simulink model "ecualizador"  (R2017b)
settings: Solver=VariableStepAuto  StartTime=0.0  StopTime=3  RelTol=1e-3
values from neighbouring files (symbols this model uses):
  ganancia = [.001 4 8 2 .1]    [DSP4.m]
  ts = 11025    [DSP4.m]
libraries: dspvision x1
settings Model: Creator=Agustin  LastModifiedBy=Agustin

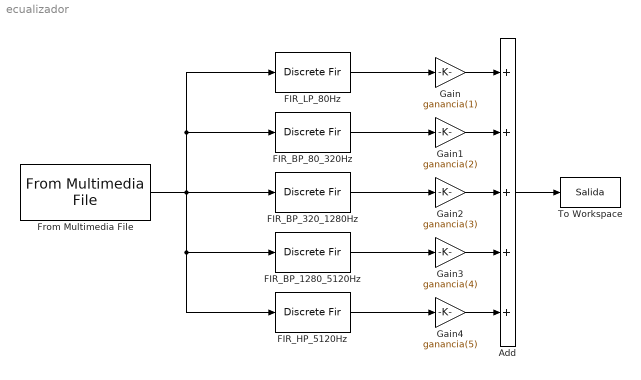
== system ecualizador ==
  Add : Sum  Inputs=+++++
  FIR_BP_1280_5120Hz : DiscreteFir  Tag=BlockMethodSubSystem  Coefficients=[-6.33540936235722367e-05 0.00195654270160462588 -4.01545452605399819e-05 0.00212945592350992276 -0.00285797352861382739 0.000192733862020878858 -0.00635868238869501546 0.00104177495203475841 -0.00246690417021121124 0.00822982232945761866 0.00663127303390260558 0.00720161481872818015 0.0036235549914843063 -0.0160254810773749479 -0.00644133758605169252 -0.0354313467654868985 0.0162538806667236642 -0.0169878821534266526 0.0727785965575659527 -0.00137886733993559853 0.0802568846706619293 -0.0750914551527820662 -0.0198348370109410477 -0.223435374456706137 -0.140838210653331991 0.695680638093415515 -0.140838210653331991 -0.223435374456706137 -0.0198348370109410477 -0.0750914551527820662 0.0802568846706619293 -0.00137886733993559853 0.0727785965575659527 -0.0169878821534266526 0.0162538806667236642 -0.0354313467654868985 -0.00644133758605169252 -0.0160254810773749479 0.0036235549914843063 0.00720161481872818015 0.00663127303390260558 0.00822982232945761866 -0.00246690417021121124 0.00104177495203475841 -0.00635868238869501546 0.000192733862020878858 -0.00285797352861382739 0.00212945592350992276 -4.01545452605399819e-05 0.00195654270160462588 -6.33540936235722367e-05]  InputProcessing=Columns as channels (frame based)  SampleTime=ts
  FIR_BP_320_1280Hz : DiscreteFir  Tag=BlockMethodSubSystem  Coefficients=[0.000419942512208930948 -3.28988295900055057e-05 -1.08715141066685234e-05 0.000698158881007576726 0.00209982001039358494 0.00368828009137740862 0.00437745590019822991 0.00294020690183505054 -0.00112851569328516698 -0.00684304173297955315 -0.0117374599789034622 -0.0130100060708184962 -0.00942737497665724691 -0.00291200710251219696 0.00142417065446380302 -0.00261072713857117382 -0.0186716075625321248 -0.044528875633302753 -0.0710778113878306611 -0.084908586891173865 -0.0738699802862342741 -0.0332917571410572821 0.0302207698048555275 0.0996866081926109926 0.153492724260163749 0.173735970087244396 0.153492724260163749 0.0996866081926109926 0.0302207698048555275 -0.0332917571410572821 -0.0738699802862342741 -0.084908586891173865 -0.0710778113878306611 -0.044528875633302753 -0.0186716075625321248 -0.00261072713857117382 0.00142417065446380302 -0.00291200710251219696 -0.00942737497665724691 -0.0130100060708184962 -0.0117374599789034622 -0.00684304173297955315 -0.00112851569328516698 0.00294020690183505054 0.00437745590019822991 0.00368828009137740862 0.00209982001039358494 0.000698158881007576726 -1.08715141066685234e-05 -3.28988295900055057e-05 0.000419942512208930948]  InputProcessing=Columns as channels (frame based)  SampleTime=ts
  FIR_BP_80_320Hz : DiscreteFir  Tag=BlockMethodSubSystem  Coefficients=[-0.00334531967217268104 -0.00351971885205419914 -0.00392813756457967289 -0.00452322525656722024 -0.00521978418872912249 -0.00589804359324740384 -0.00641026710657543238 -0.00659034250564381838 -0.00626574065394652508 -0.00527100932474330788 -0.00346180649641677574 -0.00072839160035881507 0.00299250896620734379 0.00770846163075225316 0.0133655445192406037 0.0198466230531161025 0.0269739906190492561 0.0345163619960699164 0.0421998798339282832 0.0497224859255611523 0.056770743735437057 0.0630379979484618491 0.0682426371445713775 0.0721451973109596828 0.0745631099123155588 0.0753820543913198554 0.0745631099123155588 0.0721451973109596828 0.0682426371445713775 0.0630379979484618491 0.056770743735437057 0.0497224859255611523 0.0421998798339282832 0.0345163619960699164 0.0269739906190492561 0.0198466230531161025 0.0133655445192406037 0.00770846163075225316 0.00299250896620734379 -0.00072839160035881507 -0.00346180649641677574 -0.00527100932474330788 -0.00626574065394652508 -0.00659034250564381838 -0.00641026710657543238 -0.00589804359324740384 -0.00521978418872912249 -0.00452322525656722024 -0.00392813756457967289 -0.00351971885205419914 -0.00334531967217268104]  InputProcessing=Columns as channels (frame based)  SampleTime=ts
  FIR_HP_5120Hz : DiscreteFir  Tag=BlockMethodSubSystem  Coefficients=[0.000648812761299368836 -0.000878383034572156819 0.00118621412166401837 -0.00158874360279032687 0.00207370969390318662 -0.00259433790109791802 0.00306729493039224104 -0.00337501186142079648 0.00337252739331047723 -0.00289851122739075671 0.00178964882312739808 0.000102846325584098864 -0.00289613146419001859 0.00665974099465227714 -0.011402386565635159 0.0170630529167427672 -0.0235075474141580656 0.0305311870551178977 -0.037867746896806706 0.045204202556027695 -0.0522002351697144762 0.0585109869196535209 -0.0638112083038572669 0.0678187614763474389 -0.0703154572565899 0.0711634080717828271 -0.0703154572565899 0.0678187614763474389 -0.0638112083038572669 0.0585109869196535209 -0.0522002351697144762 0.045204202556027695 -0.037867746896806706 0.0305311870551178977 -0.0235075474141580656 0.0170630529167427672 -0.011402386565635159 0.00665974099465227714 -0.00289613146419001859 0.000102846325584098864 0.00178964882312739808 -0.00289851122739075671 0.00337252739331047723 -0.00337501186142079648 0.00306729493039224104 -0.00259433790109791802 0.00207370969390318662 -0.00158874360279032687 0.00118621412166401837 -0.000878383034572156819 0.000648812761299368836]  InputProcessing=Columns as channels (frame based)  SampleTime=ts
  FIR_LP_80Hz : DiscreteFir  Tag=BlockMethodSubSystem  Coefficients=[0.00243875513785524016 0.002597139754945806 0.00298564026125039232 0.00361008381188816004 0.0044714984030764281 0.00556597304821202388 0.00688462524133961942 0.00841367810096847052 0.0101346470421464097 0.0120246332572812222 0.0140567187587707591 0.0162004553108716746 0.0184224373141124685 0.0206869466590471791 0.0229566557883360417 0.0251933737417906894 0.0273588188454260556 0.0294154009715796513 0.0313269959624674563 0.0330596948841094945 0.034582511261351874 0.0358680303276880871 0.03689298558588823 0.0376387495878988121 0.038091727767259817 0.0382436463488761147 0.038091727767259817 0.0376387495878988121 0.03689298558588823 0.0358680303276880871 0.034582511261351874 0.0330596948841094945 0.0313269959624674563 0.0294154009715796513 0.0273588188454260556 0.0251933737417906894 0.0229566557883360417 0.0206869466590471791 0.0184224373141124685 0.0162004553108716746 0.0140567187587707591 0.0120246332572812222 0.0101346470421464097 0.00841367810096847052 0.00688462524133961942 0.00556597304821202388 0.0044714984030764281 0.00361008381188816004 0.00298564026125039232 0.002597139754945806 0.00243875513785524016]  InputProcessing=Columns as channels (frame based)  SampleTime=ts
  From Multimedia File : dspvision/From Multimedia File  inputFilename=..\DSP3\Perro.wav  loop=on  numPlays=inf  outputStreams=Audio only  videoDataType=single  audioDataType=double  inheritSampleTime=on  userDefinedSampleTime=1/30  noAudioOutput=off  isIntensityVideo=off  fourcc=RGB  colorVideoFormat=Separate color signals  outputEOF=off  dataOrg=Column-major  audioFrameSize=1024  computeAudioFrameSize=off  outSamplingMode=Sample based
      settings: SourceProductBaseCode=VP
  Gain : Gain  Gain=ganancia(1)
  Gain1 : Gain  Gain=ganancia(2)
  Gain2 : Gain  Gain=ganancia(3)
  Gain3 : Gain  Gain=ganancia(4)
  Gain4 : Gain  Gain=ganancia(5)
  To Workspace : ToWorkspace  VariableName=Salida  SaveFormat=Timeseries  SampleTime=-1
  wires:
  FIR_BP_320_1280Hz/1 -> Gain2/1
  FIR_BP_1280_5120Hz/1 -> Gain3/1
  FIR_HP_5120Hz/1 -> Gain4/1
  FIR_BP_80_320Hz/1 -> Gain1/1
  FIR_LP_80Hz/1 -> Gain/1
  Gain/1 -> Add/1
  Gain1/1 -> Add/2
  Gain2/1 -> Add/3
  Gain3/1 -> Add/4
  Gain4/1 -> Add/5
  From Multimedia File/1 -> FIR_BP_1280_5120Hz/1, FIR_HP_5120Hz/1, FIR_BP_320_1280Hz/1, FIR_BP_80_320Hz/1, FIR_LP_80Hz/1
  Add/1 -> To Workspace/1
